simulink model "PubIfDecisionLSM_MDL"  (R2020b)
settings: configuration reference "DspaceConfig" (kept outside this file)
PostLoadFcn:
  | if any(exist('dsrtsu_mdlpostloadfcn', 'file') ~= 0), dsrtsu_mdlpostloadfcn('Execute', bdroot); end
InitFcn:
  | , if any(exist('rtifpga_mdlclblib', 'file') ~= 0), rtifpga_mdlclblib('Init', bdroot); end,
  | , if any(exist('dsmpb_private', 'file') ~= 0), dsmpb_private('dsmpb_mdlclblib', 'Init', bdroot); end,
values from neighbouring files (symbols this model uses):
  P_LSM_ALC_Enable = 0.0    [LSM_Parameter.sldd]
  P_LSM_AwayEdge_offset = 0.1    [LSM_Parameter.sldd]
  P_LSM_CentValidErr = 1.0    [LSM_Parameter.sldd]
  P_LSM_DOP_C0_EN_Limit = 0.8    [LSM_Parameter.sldd]
  P_LSM_DOP_C0_out_Limit = 2.0    [LSM_Parameter.sldd]
  P_LSM_DOP_C1_EN_Limit : value not decoded    [LSM_Parameter.sldd]
  P_LSM_DOP_C1_out_Limit : value not decoded    [LSM_Parameter.sldd]
  P_LSM_DOP_C1AndC2_Lim_X : value not decoded    [LSM_Parameter.sldd]
  P_LSM_DOP_C2_EN_Limit : value not decoded    [LSM_Parameter.sldd]
  P_LSM_DOP_C2_out_Limit : value not decoded    [LSM_Parameter.sldd]
  P_LSM_DOP_In_Pre2Dop_Dis = 1.0    [LSM_Parameter.sldd]
  P_LSM_DOP_Out_Pre2Dop_Dis = 2.0    [LSM_Parameter.sldd]
  P_LSM_DOP_PreDis_X : value not decoded    [LSM_Parameter.sldd]
  P_LSM_DOP_PreDis_Y : value not decoded    [LSM_Parameter.sldd]
  P_LSM_DOPEnableSW = 1.0    [LSM_Parameter.sldd]
  P_LSM_DOPValid_CheckTime = 0.06    [LSM_Parameter.sldd]
  P_LSM_DoubleLine_Curr2Cent_Dislimit = 0.5    [LSM_Parameter.sldd]
  P_LSM_DoubleLine_Dop2Cent_Dislimit = 0.5    [LSM_Parameter.sldd]
  P_LSM_DoubleLine_DOPOut_C1 : value not decoded    [LSM_Parameter.sldd]
  P_LSM_DoubleLine_Pre2Cent_Dislimit = 1.0    [LSM_Parameter.sldd]
  P_LSM_Error_Limit = 0.5    [LSM_Parameter.sldd]
  P_LSM_IFV2CenterAxis = 0.0    [LSM_Parameter.sldd]
  P_LSM_IFV2RearAxis = 0.0    [LSM_Parameter.sldd]
  P_LSM_Line2Edge_limit = 0.5    [LSM_Parameter.sldd]
  P_LSM_Line_Error = 0.1    [LSM_Parameter.sldd]
  P_LSM_LineSTD_Limit = 0.15    [LSM_Parameter.sldd]
  P_LSM_NOH_Switch = 0.0    [LSM_Parameter.sldd]
  P_LSM_OTL_C0_Factor = 1.0    [LSM_Parameter.sldd]
  P_LSM_OTL_C1_Factor = 0.5    [LSM_Parameter.sldd]
  P_LSM_OTL_C2_Factor = 0.5    [LSM_Parameter.sldd]
  P_LSM_Pre2OnlyLineDis = 5.0    [LSM_Parameter.sldd]
  P_LSM_Pre_t = 0.0    [LSM_Parameter.sldd]
  P_LSM_SingleLine_Cent2Edge_Dislimit = 100.0    [LSM_Parameter.sldd]
  P_LSM_SingleLine_Curr2Cent_Dislimit = 0.2    [LSM_Parameter.sldd]
  P_LSM_SingleLine_Dop2Cent_Dislimit = 0.2    [LSM_Parameter.sldd]
  P_LSM_SingleLine_DOPOut_C1 : value not decoded    [LSM_Parameter.sldd]
  P_LSM_SingleLine_Pre2Cent_Dislimit = 0.5    [LSM_Parameter.sldd]
  P_LSM_TJALimitSpd = 60.0    [LSM_Parameter.sldd]
undefined symbols (not defined in the file or in its folder): P_lCS_IFV2CenterAxis, P_LCS_IFV2RearAxis, P_LSM_EntryEdge_offset, P_LSM_EntryLnChngEnSwitch, P_LSM_EntryVanishDis, P_LSM_LinetLostTime, P_LSM_LineWijCal_C12, P_LSM_LineWijCal_C13, P_LSM_MapValid_ErrorSwitch, P_LSM_PosLineLcFac, P_LSM_SpdLim_Stub_Spd, P_LSM_SpdLim_StubLength, P_LSM_SpdTurnAlarm
libraries: simulink x324, TrueDurationTime x11
(part 6 of 25)

== system PubIfDecisionLSM_MDL/Subsystem1/TargetLineCalc_20ms2/DetectChange ==
  In1 : Inport
  Relational Operator1 : RelationalOperator  Operator=~=  OutDataTypeStr=boolean  RndMeth=Simplest
  Unit Delay68 : UnitDelay  SampleTime=-1  HasFrameUpgradeWarning=on
  Out1 : Outport
  wires:
  Relational Operator1/1 -> Out1/1
  In1/1 -> Relational Operator1/1, Unit Delay68/1
  Unit Delay68/1 -> Relational Operator1/2

== system PubIfDecisionLSM_MDL/Subsystem1/TargetLineCalc_20ms2/DetectChange1 ==
  In1 : Inport
  Relational Operator1 : RelationalOperator  Operator=~=  OutDataTypeStr=boolean  RndMeth=Simplest
  Unit Delay68 : UnitDelay  SampleTime=-1  HasFrameUpgradeWarning=on
  Out1 : Outport
  wires:
  Unit Delay68/1 -> Relational Operator1/2
  In1/1 -> Unit Delay68/1, Relational Operator1/1
  Relational Operator1/1 -> Out1/1

== system PubIfDecisionLSM_MDL/Subsystem1/TargetLineCalc_20ms2/DetectChange2 ==
  In1 : Inport
  Relational Operator1 : RelationalOperator  Operator=~=  OutDataTypeStr=boolean  RndMeth=Simplest
  Unit Delay68 : UnitDelay  SampleTime=-1  HasFrameUpgradeWarning=on
  Out1 : Outport
  wires:
  Relational Operator1/1 -> Out1/1
  In1/1 -> Relational Operator1/1, Unit Delay68/1
  Unit Delay68/1 -> Relational Operator1/2

== system PubIfDecisionLSM_MDL/Subsystem1/TargetLineCalc_20ms2/Simulink Function ==
  f : TriggerPort  TriggerType=function-call  IsSimulinkFunction=on  FunctionName=f  FunctionVisibility=scoped  VariantControl=(inherit)
  Constant4 : Constant  Value=P_LCS_IFV2RearAxis  OutDataTypeStr=single
  Constant5 : Constant  Value=P_lCS_IFV2CenterAxis  OutDataTypeStr=single
  MATLAB Function3 : MATLAB Function  TreatAsAtomicUnit=on
  A0 : ArgIn  DisableCoverage=on  OutDataTypeStr=single  ArgumentName=A0
  A1 : ArgIn  DisableCoverage=on  Port=2  OutDataTypeStr=single  ArgumentName=A1
  A2 : ArgIn  DisableCoverage=on  Port=3  OutDataTypeStr=single  ArgumentName=A2
  A3 : ArgIn  DisableCoverage=on  Port=4  OutDataTypeStr=single  ArgumentName=A3
  Range_min : ArgIn  DisableCoverage=on  Port=5  OutDataTypeStr=single  ArgumentName=Range_min
  Range_max : ArgIn  DisableCoverage=on  Port=6  OutDataTypeStr=single  ArgumentName=Range_max
  a0 : ArgOut  DisableCoverage=on  OutDataTypeStr=single  ArgumentName=a0
  a1 : ArgOut  DisableCoverage=on  Port=2  OutDataTypeStr=single  ArgumentName=a1
  a2 : ArgOut  DisableCoverage=on  Port=3  OutDataTypeStr=single  ArgumentName=a2
  a3 : ArgOut  DisableCoverage=on  Port=4  OutDataTypeStr=single  ArgumentName=a3
  Rmin : ArgOut  DisableCoverage=on  Port=5  OutDataTypeStr=single  ArgumentName=Rmin
  Rmax : ArgOut  DisableCoverage=on  Port=6  OutDataTypeStr=single  ArgumentName=Rmax
  wires:
  MATLAB Function3/6(Rmax) -> Rmax/1  "Rmax"
  MATLAB Function3/5(Rmin) -> Rmin/1  "Rmin"
  MATLAB Function3/4(a3) -> a3/1  "A3"
  MATLAB Function3/3(a2) -> a2/1  "A2"
  MATLAB Function3/2(a1) -> a1/1  "A1"
  MATLAB Function3/1(a0) -> a0/1  "A0"
  Range_max/1 -> MATLAB Function3/8(Range_max)
  Range_min/1 -> MATLAB Function3/7(Range_min)
  A3/1 -> MATLAB Function3/6(A3)
  A2/1 -> MATLAB Function3/5(A2)
  A1/1 -> MATLAB Function3/4(A1)
  A0/1 -> MATLAB Function3/3(A0)
  Constant5/1 -> MATLAB Function3/2(IFV2CenterAxis)
  Constant4/1 -> MATLAB Function3/1(IFV2RearAxis)

== system PubIfDecisionLSM_MDL/Subsystem1/TargetLineCalc_20ms2/Subsystem ==
  In1 : Inport
  Add : Sum  OutDataTypeStr=single
  Constant8 : Constant  Value=1.3  OutDataTypeStr=single
  Gain3 : Gain  Gain=3.6
  Gain4 : Gain  Gain=1.03
  Product : Product
  Sum : Sum  Inputs=|++
  preDisMinTable : Lookup_n-D  NumberOfTableDimensions=1  BreakpointsForDimension1=[0 5 10 15 20 25 30 35 40 60 80 90 100 110 120 140]  Table=[8 9 10 11 12 13 14 15 17 22 28 31 35 38 42 49]  ExtrapMethod=Clip  InternalRulePriority=Speed  RndMeth=Simplest  InputSameDT=on
  tDeltaEpsTable : Lookup_n-D  NumberOfTableDimensions=1  BreakpointsForDimension1=[0 5 10 15 20 25 30 35 40 60 80 90 100 110 120 140]  Table=[0.8 0.8 0.77803 0.75258 0.71864 0.65924 0.5447 0.45773 0.38348 0.2 0.2 0.2 0.20106 0.2 0.2 0.2]  ExtrapMethod=Clip  InternalRulePriority=Speed  RndMeth=Simplest  InputSameDT=on
  preDis : Outport
  wires:
  Product/1 -> Add/2
  Gain4/1 -> Sum/1
  preDisMinTable/1 -> Add/1
  Sum/1 -> preDisMinTable/1, tDeltaEpsTable/1
  Add/1 -> preDis/1
  Constant8/1 -> Sum/2
  tDeltaEpsTable/1 -> Product/1
  Gain3/1 -> Gain4/1
  In1/1 -> Gain3/1, Product/2
